simulink model "DeteccionPulsos"  (R2020a)
settings: Solver=FixedStepDiscrete  StartTime=0.0  StopTime=inf  FixedStep=0.1  RelTol=1e-3  EnableMultiTasking=on
libraries: simulink x2, arduinolib x2
settings Model: SILPILModeSetting=veronly  ExtModeTrigDuration=2  Creator=amaisinc  LastModifiedBy=amaisinc
settings OptimizationCC: EnhancedBackFolding=on  PassReuseOutputArgsAs=Individual arguments  ZeroExternalMemoryAtStartup=off  ZeroInternalMemoryAtStartup=off  MaxStackSize=64  OptimizeBlockOrder=speed  DifferentSizesBufferReuse=on  OptimizationCustomize=off  EfficientTunableParamExpr=on
settings DebuggingCC: ParameterTunabilityLossMsg=error
settings HardwareCC: ProdBitPerInt=16  ProdBitPerPointer=16  ProdBitPerSizeT=16  ProdBitPerPtrDiffT=16  ProdLargestAtomicFloat=None  ProdWordSize=8  ProdHWDeviceType=Atmel->AVR
settings SFSimCC: MATLABDynamicMemAlloc=off
settings RTWCC: SystemTargetFile=ert.tlc  HardwareBoard=Arduino Uno  TLCOptions=-aInlineSetEventsForThisBaseRateFcn=TLC_FALSE -aSuppressMultiTaskScheduler=TLC_FALSE -aRateBasedStepFcn=1  TemplateMakefile=ert_default_tmf  Toolchain=Arduino AVR  BuildConfiguration=Faster Runs
settings CodeAppCC: ForceParamTrailComments=on  IgnoreCustomStorageClasses=off  OperatorAnnotations=on  SimulinkDataObjDesc=on  SFDataObjDesc=on  InsertBlockDesc=on
settings ERTTargetCC: SupportContinuousTime=on  SupportVariableSizeSignals=on  ExtModeStaticAllocSize=250

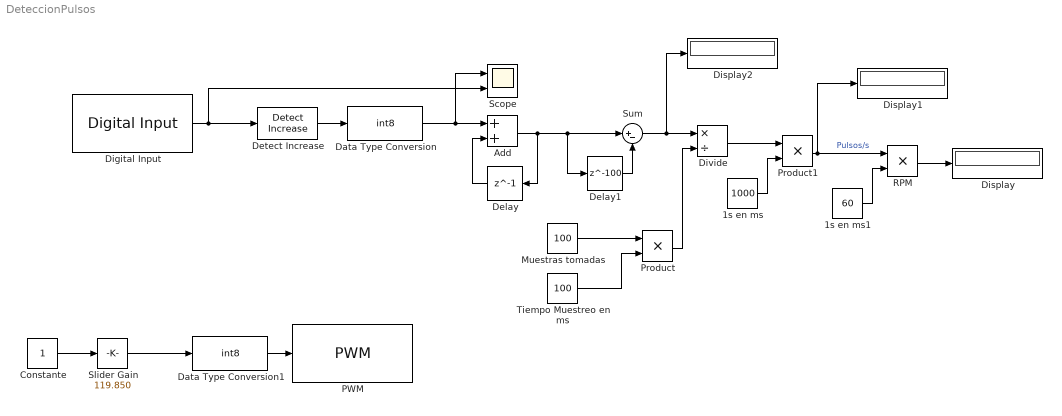
== system DeteccionPulsos ==
  1s en ms : Constant  Value=1000
  1s en ms1 : Constant  Value=60
  Add : Sum
  Constante : Constant
  Data Type Conversion : DataTypeConversion  OutDataTypeStr=int8
  Data Type Conversion1 : DataTypeConversion  OutDataTypeStr=int8
  Delay : Delay  DelayLength=1
  Delay1 : Delay  DelayLength=100
  Detect Increase : simulink/Logic and Bit Operations/Detect Increase  vinit=0.0  OutDataTypeStr=boolean
  Digital Input : arduinolib/Digital Input  pinNumber=2  Direction=input  SampleTime=-1  blockPlatform=arduino
  Display : Display
  Display1 : Display
  Display2 : Display
  Divide : Product  Inputs=*/
  Muestras tomadas : Constant  Value=100
  PWM : arduinolib/PWM  pinNumber=3  frequencyType=Specify  desiredFrequency=3921.16  achievableFrequency=3921.16
  Product : Product
  Product1 : Product
  RPM : Product
  Scope : Scope  NumInputPorts=2
  Slider Gain : simulink/Math Operations/Slider Gain  gain=119.850  low=0  high=255
  Sum : Sum  Inputs=|+-
  Tiempo Muestreo en ms : Constant  Value=100
  wires:
  Digital Input/1 -> Scope/2, Detect Increase/1
  Detect Increase/1 -> Data Type Conversion/1
  Data Type Conversion/1 -> Scope/1, Add/1
  Add/1 -> Delay1/1, Sum/1, Delay/1
  Delay/1 -> Add/2
  Delay1/1 -> Sum/2
  Sum/1 -> Display2/1, Divide/1
  Muestras tomadas/1 -> Product/1
  Tiempo Muestreo en ms/1 -> Product/2
  Product/1 -> Divide/2
  Divide/1 -> Product1/1
  1s en ms/1 -> Product1/2
  Product1/1 -> Display1/1, RPM/1  "Pulsos/s"
  1s en ms1/1 -> RPM/2
  Data Type Conversion1/1 -> PWM/1
  Slider Gain/1 -> Data Type Conversion1/1
  Constante/1 -> Slider Gain/1
  RPM/1 -> Display/1
